simulink model "simulink_drone_offline_kalman"  (R2024b)
settings: Solver=VariableStepAuto  StartTime=0.0  StopTime=10  RelTol=1e-3
values from neighbouring files (symbols this model uses):
  A = A_numeric    [offline_kalman_expanded.m]    (also in offline_kalman_kinematic.m)
  B = B_numeric    [offline_kalman_expanded.m]    (also in offline_kalman_kinematic.m = B_numeric_angular_only)
  B_kinematic = [ 0.5*dt^2  0         0 ... (first row only)    [offline_kalman_kinematic.m]
  barometer_sample_time = 1/100    (= 0.01)    [simulink_vars.m]
  barometer_variance = [0.0625]    [simulink_vars.m]
  C = C_imu    [offline_kalman_expanded.m]    (also in offline_kalman_kinematic.m = C_kinematic)
  C_barometer = [0 0 1 0 0 0 0 0 0 0 0 0 0 0 0 0 0 0]    [offline_kalman_expanded.m]
  C_gps = [1 0 0 0 0 0 0 0 0 0 0 0 0 0 0 0 0 0 ... (first row only)    [offline_kalman_expanded.m]
  g = params.g    [drone_dynamics.m]    (also in simulink_vars.m = 9.807)
  gps_sample_time = 1/20    (= 0.05)    [simulink_vars.m]
  gps_variance = 0.0025 * ones(1,3)    [simulink_vars.m]
  imu_drift = [0.0,0.0,0.0,0.00,0.00,0.00,0.0,0.0,0.0]    [simulink_vars.m]
  imu_sample_time = 1/100    (= 0.01)    [simulink_vars.m]
  imu_variance = [0.01,0.01,0.01,0.01,0.01,0.01,0.01,0.01,0.01]    [offline_kalman_kinematic.m]    (also in simulink_vars.m = [0.029,0.029,0.029,0.1225,0.1225,0.1225,0.0037,0.0037,0.0037)
  kf = round( kf, 5 )    [offline_kalman_expanded.m]    (also in offline_kalman_kinematic.m)
  kf_100 = round( kf_100, 5 )    [offline_kalman_expanded.m]
  kf_20 = round( kf_20, 5 )    [offline_kalman_expanded.m]
  params = struct()    [simulink_vars.m]
  stationary_wt = sqrt(weight/(Kt * 2))    [simulink_vars.m]
undefined symbols (not defined in the file or in its folder): process_noise
settings Model: Creator=dp271  LastModifiedBy=dp271

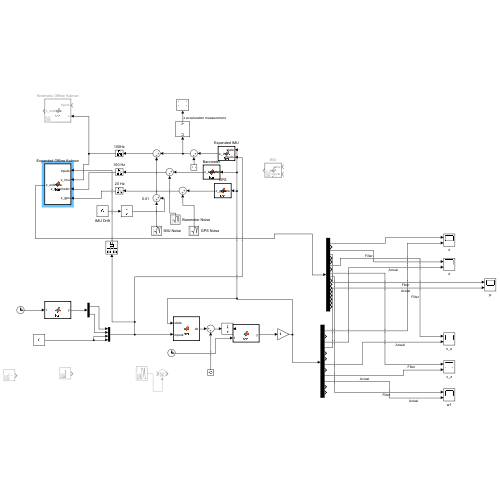
[thumbnail: Simulink's stored preview of the top-level diagram]
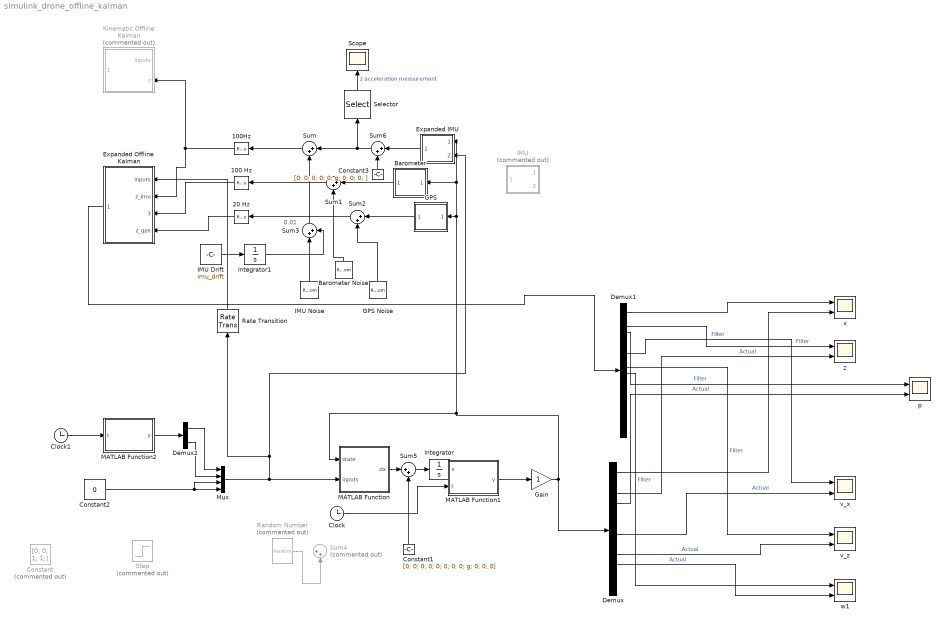
== system simulink_drone_offline_kalman ==
  note: 0.01
  " 20 Hz" : RateTransition  OutPortSampleTime=gps_sample_time
  100 Hz : RateTransition  OutPortSampleTime=barometer_sample_time
  100Hz : RateTransition  OutPortSampleTime=imu_sample_time
  Barometer : MATLAB Function  TreatAsAtomicUnit=on
  Barometer Noise : RandomNumber  Variance=barometer_variance  SampleTime=barometer_sample_time
  Clock : Clock
  Clock1 : Clock
  Constant : Constant  Commented=on  Value=[0; 0; 1; 1;]
  Constant1 : Constant  Value=[0; 0; 0; 0; 0; 0; 0; 0; g; 0; 0; 0]
  Constant2 : Constant  Value=0
  Constant3 : Constant  Value=[0; 0; 0; 0; 0; g; 0; 0; 0; ]
  Demux : Demux  Outputs=12
  Demux1 : Demux  Outputs=18
  Demux2 : Demux  Outputs=2
  Expanded IMU : MATLAB Function  TreatAsAtomicUnit=on
  Expanded Offline Kalman : MATLAB Function  TreatAsAtomicUnit=on
  GPS : MATLAB Function  TreatAsAtomicUnit=on
  GPS Noise : RandomNumber  Mean=zeros(3,1)  Variance=gps_variance  SampleTime=gps_sample_time
  Gain : Gain
  IMU : MATLAB Function  Commented=on  TreatAsAtomicUnit=on
  IMU Drift : Constant  Value=imu_drift  SampleTime=imu_sample_time
  IMU Noise : RandomNumber  Mean=zeros(9,1)  Variance=imu_variance  SampleTime=imu_sample_time
  Integrator : Integrator  InitialCondition=zeros(12,1)
  Integrator1 : Integrator  InitialCondition=zeros(9,1)
  Kinematic Offline Kalman : MATLAB Function  Commented=on  TreatAsAtomicUnit=on
  MATLAB Function : MATLAB Function  TreatAsAtomicUnit=on
  MATLAB Function1 : MATLAB Function  TreatAsAtomicUnit=on
  MATLAB Function2 : MATLAB Function  TreatAsAtomicUnit=on
  Mux : Mux
  Random Number : RandomNumber  Commented=on  Mean=zeros(12,1)  Variance=process_noise * ones(12,1)  Seed=zeros(12,1)
  Rate Transition : RateTransition  OutPortSampleTime=0.01
  Scope : Scope
  Selector : Selector  InputPortWidth=9  IndexOptions=Index vector (dialog)  Indices=[6]  OutputSizes=1
  Step : Step  Commented=on  Time=5  Before=stationary_wt  After=stationary_wt  SampleTime=0
  Sum{,1..3,5..6} (6 alike) : Sum  Inputs=|++
  Sum4 : Sum  Commented=on  Inputs=|++
  p : Scope  NumInputPorts=2
  v_x : Scope  NumInputPorts=2
  v_z : Scope  NumInputPorts=2
  w1 : Scope  NumInputPorts=2
  x : Scope  NumInputPorts=2
  z : Scope  NumInputPorts=2
  wires:
  " 20 Hz"/1 -> Expanded Offline Kalman/4(z_gps)
  Demux1/1 -> x/1
  Demux/3 -> z/2  "Actual"
  IMU Noise/1 -> Sum3/1
  Demux1/7 -> v_x/1  "Filter"
  Demux1/3 -> z/1  "Filter"
  IMU Drift/1 -> Integrator1/1
  Sum1/1 -> 100 Hz/1
  Demux/4 -> p/2  "Actual"
  Demux1/9 -> v_z/1  "Filter"
  Integrator1/1 -> Sum3/2
  Barometer Noise/1 -> Sum1/2
  Demux/7 -> v_x/2  "Actual"
  Sum2/1 -> " 20 Hz"/1
  GPS Noise/1 -> Sum2/2
  Demux/1 -> x/2
  Demux/9 -> v_z/2  "Actual"
  Sum/1 -> 100Hz/1
  Demux1/4 -> p/1  "Filter"
  Integrator/1 -> MATLAB Function1/1(x)
  Sum3/1 -> Sum/2
  GPS/1(z_gps) -> Sum2/1
  100Hz/1 -> Expanded Offline Kalman/2(z_imu), Kinematic Offline Kalman/2(z)
  Expanded Offline Kalman/1(x_estimate) -> Demux1/1
  Barometer/1(z_barometer) -> Sum1/1
  100 Hz/1 -> Expanded Offline Kalman/3(z_barometer)
  Mux/1 -> MATLAB Function/2(inputs), Expanded IMU/2(inputs), Rate Transition/1
  Selector/1 -> Scope/1  "z acceleration measurement"
  Rate Transition/1 -> Expanded Offline Kalman/1(inputs)
  Random Number/1 -> Sum4/2
  Gain/1 -> MATLAB Function/1(state), GPS/1(state), Expanded IMU/1(state), Barometer/1(state), Demux/1
  MATLAB Function1/1(y) -> Gain/1
  Clock/1 -> MATLAB Function1/2(t)
  Demux1/10 -> w1/1  "Filter"
  Demux/10 -> w1/2  "Actual"
  Clock1/1 -> MATLAB Function2/1(t)
  Demux2/1 -> Mux/1
  Demux2/2 -> Mux/2
  MATLAB Function2/1(y) -> Demux2/1
  Constant2/1 -> Mux/3, Mux/4
  Constant1/1 -> Sum5/2
  MATLAB Function/1(dx) -> Sum5/1
  Sum5/1 -> Integrator/1
  Expanded IMU/1(z_imu) -> Sum6/1
  Sum6/1 -> Sum/1, Selector/1
  Constant3/1 -> Sum6/2

== matlab function simulink_drone_offline_kalman/GPS ==
  data: state input; z_gps output
function z_gps= fcn(state)
    z_gps = gps(state);
end

== matlab function simulink_drone_offline_kalman/MATLAB Function1 ==
  data: x input; t input; y output
function y = fcn(x, t)
    % 
    % initial_angle = -7.4e-5;
    % initial_rate = 0;%-0.0279;
    % indices = [4,5,6,10,11,12]; %angles + angular rates
    % t2 = 4.1;
    % if (t > 4) && (t < t2)
    %     angle = (t2-t) * (initial_angle/(5-4));
    %     %rate = (t2-t) * (initial_rate/(5-4));
    %     x(indices) = [[angle, angle, angle];[rate, rate, rate]];
    % elseif t > t2
    %     x(indices) = 0;
    % end

    y = x;

== matlab function simulink_drone_offline_kalman/MATLAB Function2 ==
  data: t input; y output
function y = fcn(t)
    angle = 0;
    %angle = 0.1;
    y = [0;0];
    if t > 4
        y= [angle; angle]; 
    end

    % 
    % if t > 3.8 && t < 3.9
    %     y= [angle;angle];
    % elseif t > 3.9 && t < 4
    %     y= -[angle;angle];
    % else
    %     y = zeros(2,1);
    % end

== matlab function simulink_drone_offline_kalman/Kinematic Offline Kalman ==
  data: inputs input; x_estimate output; z input; A parameter; B parameter; kf parameter; C parameter; B_kinematic parameter
function x_estimate = fcn(inputs, z, A, B, kf, C, B_kinematic)
    persistent x_internal
    
    % State vectors used for derivation
    %nw = [p q u].';     % Attitude (world frame)
    %wb = [wx wy wz].';  % Angular velocity (body frame) 
    %pw = [x y z].';     % Position (world frame)
    %vb = [vx vy vz].';  % Velocity (body frame) 
    
    %SWITCHED TO WORKING IN WORLD FRAME


    dt = 0.01;
    if isempty(x_internal)
        x_internal = zeros(12,1);
    end
    
    % prediction update
    %x_pred_dot = A * x_internal + B_numeric * inputs;

    p = x_internal(4); q = x_internal(5); u = x_internal(6);     
    % Rotation matrix from body to world frame, input: roll, pitch, yaw
    R = [cos(q)*cos(u), sin(p)*sin(q)*cos(u)-cos(p)*sin(u), cos(p)*sin(q)*cos(u)+sin(p)*sin(u) ;
         cos(q)*sin(u), sin(p)*sin(q)*sin(u)+cos(p)*cos(u), cos(p)*sin(q)*sin(u)-sin(p)*cos(u) ;
         -sin(q),       sin(p)*cos(q),                      cos(p)*cos(q)                     ];

    g = 9.807;
    acc_total_world = R*z(4:6) - [0; 0; g];
    x_pred = A * x_internal + B_kinematic * acc_total_world + B * inputs; %Kinematic model
    %x_pred = x_internal + x_pred_dot;
    
    % measurement update
    x_internal = x_pred + kf * ([z(1:3); z(7:9)] - C * x_pred); %No dt here because dlqe should account for it
    
    x_estimate = x_internal;
    %x_estimate(7:9) = R * x_internal(7:9);
end

== matlab function simulink_drone_offline_kalman/MATLAB Function ==
  data: state input; inputs input; dx output; params parameter
function dx = fcn(state, inputs, params)

    dx = drone_dynamics(state, inputs, params);

end

== matlab function simulink_drone_offline_kalman/Barometer ==
  data: state input; z_barometer output
function z_barometer= fcn(state)
    z_barometer = barometer(state);
end

== matlab function simulink_drone_offline_kalman/Expanded Offline Kalman ==
  data: inputs input; z_imu input; z_barometer input; z_gps input; x_estimate output; kf_20 parameter; kf_100 parameter; params parameter; C_barometer parameter; C_gps parameter
function x_estimate = fcn(inputs, z_imu, z_barometer, z_gps, kf_20, kf_100, params, C_barometer, C_gps)
    persistent x_internal last_gps_val

    %initialises internal state estimate + last gps value
    if isempty(x_internal)
        x_internal = zeros(18,1);
    end

    if isempty(last_gps_val)
        last_gps_val = zeros(3,1);
    end

    [x_internal, last_gps_val] = kalman_filter(x_internal, last_gps_val, inputs, z_imu, z_barometer, z_gps, kf_20, kf_100, params, C_barometer, C_gps);
    
    x_estimate = x_internal;

    
    % 
    % coder.extrinsic('fprintf');
    % 
    % %initialises internal state estimate + last gps value (to detect new
    % %gps val)
    % if isempty(x_internal)
    %     x_internal = zeros(18,1);
    % end
    % 
    % if isempty(last_gps_val)
    %     last_gps_val = zeros(3,1);
    % end
    % 
    % %Check if there is a new gps value
    % gps_delta = last_gps_val - z_gps;
    % if any(gps_delta)
    %     fprintf('');
    %     %fprintf('Inputs are %f',inputs(3));
    %     %new gps data
    %     gps_present = true;
    %     last_gps_val = z_gps;
    % else
    %     % No new gps data
    %     gps_present = false;
    % end
    % 
    % %retrieves A, B, and H_imu matrices
    % [A,B, H_imu] = calc_Jacobians(x_internal, inputs);
    % 
    % % Calculates rotation matrix from body to world frame, input: roll, pitch, yaw
    % p = x_internal(4); q = x_internal(5); u = x_internal(6);     
    % R = [cos(q)*cos(u), sin(p)*sin(q)*cos(u)-cos(p)*sin(u), cos(p)*sin(q)*cos(u)+sin(p)*sin(u) ;
    %      cos(q)*sin(u), sin(p)*sin(q)*sin(u)+cos(p)*cos(u), cos(p)*sin(q)*sin(u)-sin(p)*cos(u) ;
    %      -sin(q),       sin(p)*cos(q),                      cos(p)*cos(q)                     ];
    % 
    % % Prediction update
    % g_correction = zeros(18,1);
    % g_correction(15) = -params.g*0;
    % x_pred = A * x_internal + 0.5*B * inputs + g_correction;
    % fprintf('\n\nPredicted z acceleration  = %f', x_pred(15));
    % 
    % % Convert imu measurements from body to world frame
    % zw_acc = R * z_imu(4:6);
    % z_imu = [z_imu(1:3);zw_acc;z_imu(7:9)];
    % 
    % % Measurement update
    % if gps_present
    %     C_20_calc = [H_imu; C_barometer; C_gps];
    % 
    %     z = [z_imu; z_barometer; z_gps];
    % 
    %     x_internal = x_pred + kf_20 * (z - C_20_calc * (x_pred - g_correction));
    % else
    %     C_100_calc = [H_imu; C_barometer];
    %     z = [z_imu; z_barometer];
    %     x_internal = x_pred + kf_100 * (z - C_100_calc * (x_pred - g_correction)); 
    % end
    % fprintf('\nEstimated z acceleration  = %f', x_internal(15));
    % 
    % x_estimate = x_internal;
end

== matlab function simulink_drone_offline_kalman/Expanded IMU ==
  data: state input; z_imu output; inputs input; params parameter
function z_imu = fcn(state, inputs, params)
    %% Right now I can;t use expanded_imu because that function takes in 18x1 state vector    


    % Extract States 
    % Euler Angles (Roll, Pitch, Yaw)
    p = state(4); q = state(5); u = state(6); 
    % Angular Rates (p, q, r)
    wx = state(10); wy = state(11); wz = state(12);

    % Extract control inputs
    a1 = inputs(1); a2 = inputs(2); wt1 = inputs(3); wt2 = inputs(4); % angles, rotation rates

    % Drone Constants
    m  = params.m;
    g  = params.g;
    Kt = params.Kt;
        
    % Rotation matrix from body to world frame, input: roll, pitch, yaw
    R = [cos(q)*cos(u), sin(p)*sin(q)*cos(u)-cos(p)*sin(u), cos(p)*sin(q)*cos(u)+sin(p)*sin(u) ;
         cos(q)*sin(u), sin(p)*sin(q)*sin(u)+cos(p)*cos(u), cos(p)*sin(q)*sin(u)-sin(p)*cos(u) ;
         -sin(q),       sin(p)*cos(q),                      cos(p)*cos(q)                     ];
        
    % Magnitude of force from rotor
    Ft = Kt * (wt1^2 + wt2 ^2);
    
    % Direction of gimbal
    X_force = [sin(a2) * cos(a1);
               -sin(a1);
               cos(a2) * cos(a1)];
    
    % Force from rotors
    fb = Ft * X_force;
        
    % State vectors used for derivation
    nw = [p q u].';     % Attitude (world frame)
    wb = [wx wy wz].';  % Angular velocity (body frame) 

    vb_dot = 1/m * ( fb);

    z_imu = [nw; % angular position
            vb_dot; % linear acceleration in body frame
            wb]; % angular velcity

end

== matlab function simulink_drone_offline_kalman/IMU ==
  data: state input; z_imu output; inputs input
function z_imu = fcn(state, inputs)
    z_imu = imu(state, inputs);
end
